simulink model "feedback_loop"  (Simulink 7.9)
settings: Solver=ode45  StartTime=0.0  StopTime=2000  RelTol=1e-3
settings Model: Creator=kr2112  LastModifiedBy=kr2112

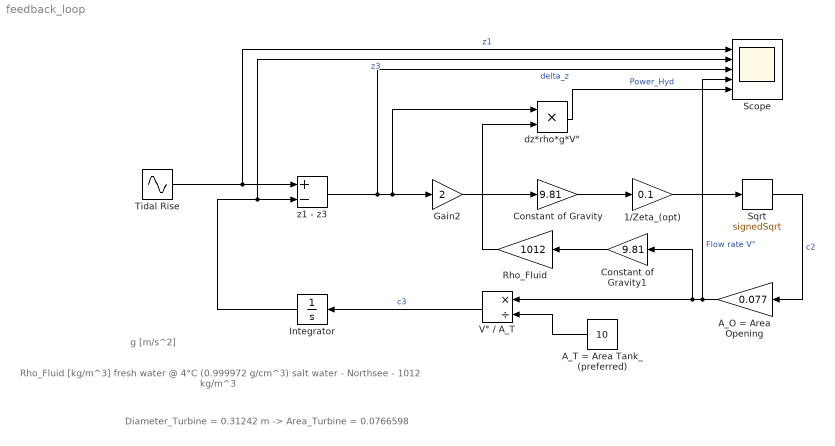
== system feedback_loop ==
  note: Rho_Fluid [kg/m^3]
      | fresh water @ 4°C (0.999972 g/cm^3)
      | salt water - Northsee - 1012 kg/m^3
  note: g [m/s^2]
  note: Diameter_Turbine = 0.31242 m -> Area_Turbine = 0.0766598
  1/Zeta_(opt) : Gain  Gain=0.1
  A_O = Area Opening : Gain  Gain=0.077
  A_T = Area Tank_(preferred) : Constant  Value=10
  Constant of Gravity : Gain  Gain=9.81
  Constant of Gravity1 : Gain  Gain=9.81
  Gain2 : Gain  Gain=2
  Integrator : Integrator
  Rho_Fluid : Gain  Gain=1012
  Scope : Scope  NumInputPorts=5
      settings: TimeRange=2000  YMin=-5~-5~-5~-5~-5  YMax=5~5~5~5~5
  Sqrt : Sqrt  Operator=signedSqrt  SaturateOnIntegerOverflow=on
  Tidal Rise : Sin  Frequency=0.0083  SampleTime=0
  V° / A_T : Product  Inputs=*/
  dz*rho*g*V° : Product  RndMeth=Zero
  z1 - z3 : Sum  Inputs=+-
  wires:
  Constant of Gravity/1 -> 1/Zeta_(opt)/1
  Sqrt/1 -> A_O = Area Opening/1  "c2"
  z1 - z3/1 -> Scope/3, dz*rho*g*V°/1, Gain2/1  "delta_z"
  Tidal Rise/1 -> z1 - z3/1, Scope/1  "z1"
  Integrator/1 -> z1 - z3/2, Scope/2  "z3"
  A_T = Area Tank_(preferred)/1 -> V° / A_T/2
  V° / A_T/1 -> Integrator/1  "c3"
  dz*rho*g*V°/1 -> Scope/5  "Power_Hyd"
  Constant of Gravity1/1 -> Rho_Fluid/1
  Rho_Fluid/1 -> dz*rho*g*V°/2
  A_O = Area Opening/1 -> V° / A_T/1, Constant of Gravity1/1, Scope/4  "Flow rate V°"
  Gain2/1 -> Constant of Gravity/1
  1/Zeta_(opt)/1 -> Sqrt/1
